simulink model "Adaptive_cascade_rov"  (Simulink 6.0)
settings: Solver=ode45  StartTime=0.0  StopTime=650  RelTol=1e-3
undefined symbols (not defined in the file): B, DQ, DQL, I, m, M, Ma, MaL, MaU, rg, sigbuilder_block, T, W, xb, xg, Xudot, yb, yg, Yvdot, zb, zg, Zwdot
libraries: simulink_extras x12, simulink x8
(part 3 of 3)

== system Adaptive_cascade_rov/inner-loop controller/inner -PI-decouple /thruster  dynamic     /thruster  alloc. /thruster  allocation control1/thruster allocation /Atomic Subsystem4 ==
  In1 : Inport  Port=1  LatchInput=off
  In2 : Inport  Port=2  LatchInput=off
  In3 : Inport  Port=3  LatchInput=off
  Enable : EnablePort
  Subtract : Sum  Inputs=+++  OutScaling=2^-10
  Out1 : Outport
  wires:
  In1/1 -> Subtract/1
  In2/1 -> Subtract/2
  In3/1 -> Subtract/3
  Subtract/1 -> Out1/1

== system Adaptive_cascade_rov/inner-loop controller/inner -PI-decouple /thruster  dynamic     /thruster  alloc. /thruster  allocation control1/thruster allocation /Atomic Subsystem5 ==
  In1 : Inport  Port=1  LatchInput=off
  In2 : Inport  Port=2  LatchInput=off
  In3 : Inport  Port=3  LatchInput=off
  Enable : EnablePort
  Subtract : Sum  Inputs=+++  OutScaling=2^-10
  Out1 : Outport
  wires:
  In1/1 -> Subtract/1
  In2/1 -> Subtract/2
  In3/1 -> Subtract/3
  Subtract/1 -> Out1/1

== system Adaptive_cascade_rov/inner-loop controller/inner -PI-decouple /thruster  dynamic     /thruster  alloc. /thruster  allocation control1/thruster allocation /Atomic Subsystem6 ==
  In1 : Inport  Port=1  LatchInput=off
  In2 : Inport  Port=2  LatchInput=off
  Enable : EnablePort
  Subtract : Sum  OutScaling=2^-10
  Out1 : Outport
  wires:
  In1/1 -> Subtract/1
  In2/1 -> Subtract/2
  Subtract/1 -> Out1/1

== system Adaptive_cascade_rov/inner-loop controller/inner -PI-decouple /thruster  dynamic     /thruster  alloc. /thruster  allocation control1/thruster allocation /Atomic Subsystem7 ==
  1 : Inport  Port=1  LatchInput=off
  2 : Inport  Port=2  LatchInput=off
  Enable : EnablePort
  Subtract : Sum  OutScaling=2^-10
  Out1 : Outport
  wires:
  1/1 -> Subtract/1
  2/1 -> Subtract/2
  Subtract/1 -> Out1/1

== system Adaptive_cascade_rov/inner-loop controller/inner -PI-decouple /thruster  dynamic     /thruster  alloc. /thruster  allocation control1/thruster allocation /Atomic Subsystem8 ==
  In2 : Inport  Port=1  LatchInput=off
  Abs : Abs
  Product1 : Product  OutDataTypeMode=double  SaturateOnIntegerOverflow=on  RndMeth=Zero
  Product5 : Product  OutDataTypeMode=double  SaturateOnIntegerOverflow=on  RndMeth=Zero
  Sign1 : Signum
  Switch1 : Switch  Threshold=1  SaturateOnIntegerOverflow=on  InputSameDT=on
  <0 : Outport
  wires:
  In2/1 -> Sign1/1, Product1/1, Abs/1
  Sign1/1 -> Switch1/2, Product1/2, Product5/1
  Product1/1 -> Switch1/1
  Product5/1 -> Switch1/3
  Switch1/1 -> <0/1
  Abs/1 -> Product5/2

== system Adaptive_cascade_rov/inner-loop controller/inner -backstepping/thruster  dynamic     /thruster  alloc. /thruster  allocation control1/thruster allocation /Atomic Subsystem1 ==
  In2 : Inport  Port=1  LatchInput=off
  Abs : Abs
  Product1 : Product  OutDataTypeMode=double  SaturateOnIntegerOverflow=on  RndMeth=Zero
  Product5 : Product  OutDataTypeMode=double  SaturateOnIntegerOverflow=on  RndMeth=Zero
  Sign1 : Signum
  Switch1 : Switch  Threshold=1  SaturateOnIntegerOverflow=on  InputSameDT=on
  <0 : Outport
  wires:
  Sign1/1 -> Product1/2, Product5/1, Switch1/2
  Product1/1 -> Switch1/1
  Product5/1 -> Switch1/3
  Switch1/1 -> <0/1
  In2/1 -> Sign1/1, Product1/1, Abs/1
  Abs/1 -> Product5/2

== system Adaptive_cascade_rov/inner-loop controller/inner -backstepping/thruster  dynamic     /thruster  alloc. /thruster  allocation control1/thruster allocation /Atomic Subsystem2 ==
  In2 : Inport  Port=1  LatchInput=off
  Abs : Abs
  Product1 : Product  OutDataTypeMode=double  SaturateOnIntegerOverflow=on  RndMeth=Zero
  Product5 : Product  OutDataTypeMode=double  SaturateOnIntegerOverflow=on  RndMeth=Zero
  Sign1 : Signum
  Switch1 : Switch  Threshold=1  SaturateOnIntegerOverflow=on  InputSameDT=on
  <0 : Outport
  wires:
  In2/1 -> Sign1/1, Product1/1, Abs/1
  Sign1/1 -> Switch1/2, Product1/2, Product5/1
  Product1/1 -> Switch1/1
  Product5/1 -> Switch1/3
  Switch1/1 -> <0/1
  Abs/1 -> Product5/2

== system Adaptive_cascade_rov/inner-loop controller/inner -backstepping/thruster  dynamic     /thruster  alloc. /thruster  allocation control1/thruster allocation /Atomic Subsystem3 ==
  In2 : Inport  Port=1  LatchInput=off
  Abs : Abs
  Product1 : Product  OutDataTypeMode=double  SaturateOnIntegerOverflow=on  RndMeth=Zero
  Product5 : Product  OutDataTypeMode=double  SaturateOnIntegerOverflow=on  RndMeth=Zero
  Sign1 : Signum
  Switch1 : Switch  Threshold=1  SaturateOnIntegerOverflow=on  InputSameDT=on
  <0 : Outport
  wires:
  Sign1/1 -> Switch1/2, Product1/2, Product5/1
  Product1/1 -> Switch1/1
  Product5/1 -> Switch1/3
  Switch1/1 -> <0/1
  In2/1 -> Sign1/1, Product1/1, Abs/1
  Abs/1 -> Product5/2

== system Adaptive_cascade_rov/inner-loop controller/inner -backstepping/thruster  dynamic     /thruster  alloc. /thruster  allocation control1/thruster allocation /Atomic Subsystem4 ==
  In1 : Inport  Port=1  LatchInput=off
  In2 : Inport  Port=2  LatchInput=off
  In3 : Inport  Port=3  LatchInput=off
  Enable : EnablePort
  Subtract : Sum  Inputs=+++  OutScaling=2^-10
  Out1 : Outport
  wires:
  In1/1 -> Subtract/1
  In2/1 -> Subtract/2
  In3/1 -> Subtract/3
  Subtract/1 -> Out1/1

== system Adaptive_cascade_rov/inner-loop controller/inner -backstepping/thruster  dynamic     /thruster  alloc. /thruster  allocation control1/thruster allocation /Atomic Subsystem5 ==
  In1 : Inport  Port=1  LatchInput=off
  In2 : Inport  Port=2  LatchInput=off
  In3 : Inport  Port=3  LatchInput=off
  Enable : EnablePort
  Subtract : Sum  Inputs=+++  OutScaling=2^-10
  Out1 : Outport
  wires:
  In1/1 -> Subtract/1
  In2/1 -> Subtract/2
  In3/1 -> Subtract/3
  Subtract/1 -> Out1/1

== system Adaptive_cascade_rov/inner-loop controller/inner -backstepping/thruster  dynamic     /thruster  alloc. /thruster  allocation control1/thruster allocation /Atomic Subsystem6 ==
  In1 : Inport  Port=1  LatchInput=off
  In2 : Inport  Port=2  LatchInput=off
  Enable : EnablePort
  Subtract : Sum  OutScaling=2^-10
  Out1 : Outport
  wires:
  In1/1 -> Subtract/1
  In2/1 -> Subtract/2
  Subtract/1 -> Out1/1

== system Adaptive_cascade_rov/inner-loop controller/inner -backstepping/thruster  dynamic     /thruster  alloc. /thruster  allocation control1/thruster allocation /Atomic Subsystem7 ==
  1 : Inport  Port=1  LatchInput=off
  2 : Inport  Port=2  LatchInput=off
  Enable : EnablePort
  Subtract : Sum  OutScaling=2^-10
  Out1 : Outport
  wires:
  1/1 -> Subtract/1
  2/1 -> Subtract/2
  Subtract/1 -> Out1/1

== system Adaptive_cascade_rov/inner-loop controller/inner -backstepping/thruster  dynamic     /thruster  alloc. /thruster  allocation control1/thruster allocation /Atomic Subsystem8 ==
  In2 : Inport  Port=1  LatchInput=off
  Abs : Abs
  Product1 : Product  OutDataTypeMode=double  SaturateOnIntegerOverflow=on  RndMeth=Zero
  Product5 : Product  OutDataTypeMode=double  SaturateOnIntegerOverflow=on  RndMeth=Zero
  Sign1 : Signum
  Switch1 : Switch  Threshold=1  SaturateOnIntegerOverflow=on  InputSameDT=on
  <0 : Outport
  wires:
  In2/1 -> Sign1/1, Product1/1, Abs/1
  Sign1/1 -> Switch1/2, Product1/2, Product5/1
  Product1/1 -> Switch1/1
  Product5/1 -> Switch1/3
  Switch1/1 -> <0/1
  Abs/1 -> Product5/2

== system Adaptive_cascade_rov/inner-loop controller/inner-P/thruster  dynamic     /thruster  alloc. /thruster  allocation control1/thruster allocation /Atomic Subsystem1 ==
  In2 : Inport  Port=1  LatchInput=off
  Abs : Abs
  Product1 : Product  OutDataTypeMode=double  SaturateOnIntegerOverflow=on  RndMeth=Zero
  Product5 : Product  OutDataTypeMode=double  SaturateOnIntegerOverflow=on  RndMeth=Zero
  Sign1 : Signum
  Switch1 : Switch  Threshold=1  SaturateOnIntegerOverflow=on  InputSameDT=on
  <0 : Outport
  wires:
  Sign1/1 -> Product1/2, Product5/1, Switch1/2
  Product1/1 -> Switch1/1
  Product5/1 -> Switch1/3
  Switch1/1 -> <0/1
  In2/1 -> Sign1/1, Product1/1, Abs/1
  Abs/1 -> Product5/2

== system Adaptive_cascade_rov/inner-loop controller/inner-P/thruster  dynamic     /thruster  alloc. /thruster  allocation control1/thruster allocation /Atomic Subsystem2 ==
  In2 : Inport  Port=1  LatchInput=off
  Abs : Abs
  Product1 : Product  OutDataTypeMode=double  SaturateOnIntegerOverflow=on  RndMeth=Zero
  Product5 : Product  OutDataTypeMode=double  SaturateOnIntegerOverflow=on  RndMeth=Zero
  Sign1 : Signum
  Switch1 : Switch  Threshold=1  SaturateOnIntegerOverflow=on  InputSameDT=on
  <0 : Outport
  wires:
  In2/1 -> Sign1/1, Product1/1, Abs/1
  Sign1/1 -> Switch1/2, Product1/2, Product5/1
  Product1/1 -> Switch1/1
  Product5/1 -> Switch1/3
  Switch1/1 -> <0/1
  Abs/1 -> Product5/2

== system Adaptive_cascade_rov/inner-loop controller/inner-P/thruster  dynamic     /thruster  alloc. /thruster  allocation control1/thruster allocation /Atomic Subsystem3 ==
  In2 : Inport  Port=1  LatchInput=off
  Abs : Abs
  Product1 : Product  OutDataTypeMode=double  SaturateOnIntegerOverflow=on  RndMeth=Zero
  Product5 : Product  OutDataTypeMode=double  SaturateOnIntegerOverflow=on  RndMeth=Zero
  Sign1 : Signum
  Switch1 : Switch  Threshold=1  SaturateOnIntegerOverflow=on  InputSameDT=on
  <0 : Outport
  wires:
  Sign1/1 -> Switch1/2, Product1/2, Product5/1
  Product1/1 -> Switch1/1
  Product5/1 -> Switch1/3
  Switch1/1 -> <0/1
  In2/1 -> Sign1/1, Product1/1, Abs/1
  Abs/1 -> Product5/2

== system Adaptive_cascade_rov/inner-loop controller/inner-P/thruster  dynamic     /thruster  alloc. /thruster  allocation control1/thruster allocation /Atomic Subsystem4 ==
  In1 : Inport  Port=1  LatchInput=off
  In2 : Inport  Port=2  LatchInput=off
  In3 : Inport  Port=3  LatchInput=off
  Enable : EnablePort
  Subtract : Sum  Inputs=+++  OutScaling=2^-10
  Out1 : Outport
  wires:
  In1/1 -> Subtract/1
  In2/1 -> Subtract/2
  In3/1 -> Subtract/3
  Subtract/1 -> Out1/1

== system Adaptive_cascade_rov/inner-loop controller/inner-P/thruster  dynamic     /thruster  alloc. /thruster  allocation control1/thruster allocation /Atomic Subsystem5 ==
  In1 : Inport  Port=1  LatchInput=off
  In2 : Inport  Port=2  LatchInput=off
  In3 : Inport  Port=3  LatchInput=off
  Enable : EnablePort
  Subtract : Sum  Inputs=+++  OutScaling=2^-10
  Out1 : Outport
  wires:
  In1/1 -> Subtract/1
  In2/1 -> Subtract/2
  In3/1 -> Subtract/3
  Subtract/1 -> Out1/1

== system Adaptive_cascade_rov/inner-loop controller/inner-P/thruster  dynamic     /thruster  alloc. /thruster  allocation control1/thruster allocation /Atomic Subsystem6 ==
  In1 : Inport  Port=1  LatchInput=off
  In2 : Inport  Port=2  LatchInput=off
  Enable : EnablePort
  Subtract : Sum  OutScaling=2^-10
  Out1 : Outport
  wires:
  In1/1 -> Subtract/1
  In2/1 -> Subtract/2
  Subtract/1 -> Out1/1

== system Adaptive_cascade_rov/inner-loop controller/inner-P/thruster  dynamic     /thruster  alloc. /thruster  allocation control1/thruster allocation /Atomic Subsystem7 ==
  1 : Inport  Port=1  LatchInput=off
  2 : Inport  Port=2  LatchInput=off
  Enable : EnablePort
  Subtract : Sum  OutScaling=2^-10
  Out1 : Outport
  wires:
  1/1 -> Subtract/1
  2/1 -> Subtract/2
  Subtract/1 -> Out1/1

== system Adaptive_cascade_rov/inner-loop controller/inner-P/thruster  dynamic     /thruster  alloc. /thruster  allocation control1/thruster allocation /Atomic Subsystem8 ==
  In2 : Inport  Port=1  LatchInput=off
  Abs : Abs
  Product1 : Product  OutDataTypeMode=double  SaturateOnIntegerOverflow=on  RndMeth=Zero
  Product5 : Product  OutDataTypeMode=double  SaturateOnIntegerOverflow=on  RndMeth=Zero
  Sign1 : Signum
  Switch1 : Switch  Threshold=1  SaturateOnIntegerOverflow=on  InputSameDT=on
  <0 : Outport
  wires:
  In2/1 -> Sign1/1, Product1/1, Abs/1
  Sign1/1 -> Switch1/2, Product1/2, Product5/1
  Product1/1 -> Switch1/1
  Product5/1 -> Switch1/3
  Switch1/1 -> <0/1
  Abs/1 -> Product5/2

== system Adaptive_cascade_rov/inner-loop controller/inner-sliding/thruster  dynamic     /thruster  alloc. /thruster  allocation control1/thruster allocation /Atomic Subsystem1 ==
  In2 : Inport  Port=1  LatchInput=off
  Abs : Abs
  Product1 : Product  OutDataTypeMode=double  SaturateOnIntegerOverflow=on  RndMeth=Zero
  Product5 : Product  OutDataTypeMode=double  SaturateOnIntegerOverflow=on  RndMeth=Zero
  Sign1 : Signum
  Switch1 : Switch  Threshold=1  SaturateOnIntegerOverflow=on  InputSameDT=on
  <0 : Outport
  wires:
  Sign1/1 -> Product1/2, Product5/1, Switch1/2
  Product1/1 -> Switch1/1
  Product5/1 -> Switch1/3
  Switch1/1 -> <0/1
  In2/1 -> Sign1/1, Product1/1, Abs/1
  Abs/1 -> Product5/2

== system Adaptive_cascade_rov/inner-loop controller/inner-sliding/thruster  dynamic     /thruster  alloc. /thruster  allocation control1/thruster allocation /Atomic Subsystem2 ==
  In2 : Inport  Port=1  LatchInput=off
  Abs : Abs
  Product1 : Product  OutDataTypeMode=double  SaturateOnIntegerOverflow=on  RndMeth=Zero
  Product5 : Product  OutDataTypeMode=double  SaturateOnIntegerOverflow=on  RndMeth=Zero
  Sign1 : Signum
  Switch1 : Switch  Threshold=1  SaturateOnIntegerOverflow=on  InputSameDT=on
  <0 : Outport
  wires:
  In2/1 -> Sign1/1, Product1/1, Abs/1
  Sign1/1 -> Switch1/2, Product1/2, Product5/1
  Product1/1 -> Switch1/1
  Product5/1 -> Switch1/3
  Switch1/1 -> <0/1
  Abs/1 -> Product5/2

== system Adaptive_cascade_rov/inner-loop controller/inner-sliding/thruster  dynamic     /thruster  alloc. /thruster  allocation control1/thruster allocation /Atomic Subsystem3 ==
  In2 : Inport  Port=1  LatchInput=off
  Abs : Abs
  Product1 : Product  OutDataTypeMode=double  SaturateOnIntegerOverflow=on  RndMeth=Zero
  Product5 : Product  OutDataTypeMode=double  SaturateOnIntegerOverflow=on  RndMeth=Zero
  Sign1 : Signum
  Switch1 : Switch  Threshold=1  SaturateOnIntegerOverflow=on  InputSameDT=on
  <0 : Outport
  wires:
  Sign1/1 -> Switch1/2, Product1/2, Product5/1
  Product1/1 -> Switch1/1
  Product5/1 -> Switch1/3
  Switch1/1 -> <0/1
  In2/1 -> Sign1/1, Product1/1, Abs/1
  Abs/1 -> Product5/2

== system Adaptive_cascade_rov/inner-loop controller/inner-sliding/thruster  dynamic     /thruster  alloc. /thruster  allocation control1/thruster allocation /Atomic Subsystem4 ==
  In1 : Inport  Port=1  LatchInput=off
  In2 : Inport  Port=2  LatchInput=off
  In3 : Inport  Port=3  LatchInput=off
  Enable : EnablePort
  Subtract : Sum  Inputs=+++  OutScaling=2^-10
  Out1 : Outport
  wires:
  In1/1 -> Subtract/1
  In2/1 -> Subtract/2
  In3/1 -> Subtract/3
  Subtract/1 -> Out1/1

== system Adaptive_cascade_rov/inner-loop controller/inner-sliding/thruster  dynamic     /thruster  alloc. /thruster  allocation control1/thruster allocation /Atomic Subsystem5 ==
  In1 : Inport  Port=1  LatchInput=off
  In2 : Inport  Port=2  LatchInput=off
  In3 : Inport  Port=3  LatchInput=off
  Enable : EnablePort
  Subtract : Sum  Inputs=+++  OutScaling=2^-10
  Out1 : Outport
  wires:
  In1/1 -> Subtract/1
  In2/1 -> Subtract/2
  In3/1 -> Subtract/3
  Subtract/1 -> Out1/1

== system Adaptive_cascade_rov/inner-loop controller/inner-sliding/thruster  dynamic     /thruster  alloc. /thruster  allocation control1/thruster allocation /Atomic Subsystem6 ==
  In1 : Inport  Port=1  LatchInput=off
  In2 : Inport  Port=2  LatchInput=off
  Enable : EnablePort
  Subtract : Sum  OutScaling=2^-10
  Out1 : Outport
  wires:
  In1/1 -> Subtract/1
  In2/1 -> Subtract/2
  Subtract/1 -> Out1/1

== system Adaptive_cascade_rov/inner-loop controller/inner-sliding/thruster  dynamic     /thruster  alloc. /thruster  allocation control1/thruster allocation /Atomic Subsystem7 ==
  1 : Inport  Port=1  LatchInput=off
  2 : Inport  Port=2  LatchInput=off
  Enable : EnablePort
  Subtract : Sum  OutScaling=2^-10
  Out1 : Outport
  wires:
  1/1 -> Subtract/1
  2/1 -> Subtract/2
  Subtract/1 -> Out1/1

== system Adaptive_cascade_rov/inner-loop controller/inner-sliding/thruster  dynamic     /thruster  alloc. /thruster  allocation control1/thruster allocation /Atomic Subsystem8 ==
  In2 : Inport  Port=1  LatchInput=off
  Abs : Abs
  Product1 : Product  OutDataTypeMode=double  SaturateOnIntegerOverflow=on  RndMeth=Zero
  Product5 : Product  OutDataTypeMode=double  SaturateOnIntegerOverflow=on  RndMeth=Zero
  Sign1 : Signum
  Switch1 : Switch  Threshold=1  SaturateOnIntegerOverflow=on  InputSameDT=on
  <0 : Outport
  wires:
  In2/1 -> Sign1/1, Product1/1, Abs/1
  Sign1/1 -> Switch1/2, Product1/2, Product5/1
  Product1/1 -> Switch1/1
  Product5/1 -> Switch1/3
  Switch1/1 -> <0/1
  Abs/1 -> Product5/2
